simulink model "Advance Traction Motor and Regeneration Modeling"  (R2021a)
settings: Solver=FixedStepAuto  StartTime=0.0  StopTime=inf  FixedStep=1  RelTol=1e-3
values from neighbouring files (symbols this model uses):
  Battery_E = 24000    [Imports.m]
  BPC = 66.2    [Imports.m]
  C_SOC = Value3(:,3)    [Imports.m]
  C_V = Value3(:,2)    [Imports.m]
  Cd = 0.28    [Imports.m]
  Crf = 0.015    [Imports.m]
  Fa = 3.8056    [Imports.m]
  GR = 7.9377    [Imports.m]
  GVM = Mv+Md    (= 1710.665)    [Imports.m]
  GVW = GVM*g    (= 16781.62365)    [Imports.m]
  Ir = 0.0023    [Imports.m]
  Kemf = 0.238    [Imports.m]
  Kt = 0.195    [Imports.m]
  LSOC = 20    [Imports.m]
  M_B_R_C = M_R_C*Np    (= 66.2)    [Imports.m]
  Ns = 96    [Imports.m]
  Ra = 0.00567    [Imports.m]
  rho = 1.225    [Imports.m]
  Rw = 0.2032    [Imports.m]
  Teff = 0.89    [Imports.m]
  USOC = 80    [Imports.m]
undefined symbols (not defined in the file or in its folder): NL_M, NL_MC, NL_RM
settings Model: Creator=goodbox  LastModifiedBy=LENOVO
settings SolverCC: ShapePreserveControl=EnableAll  AlgebraicLoopSolver=TrustRegion
settings DebuggingCC: SFMachineParentedDataDiag=warning

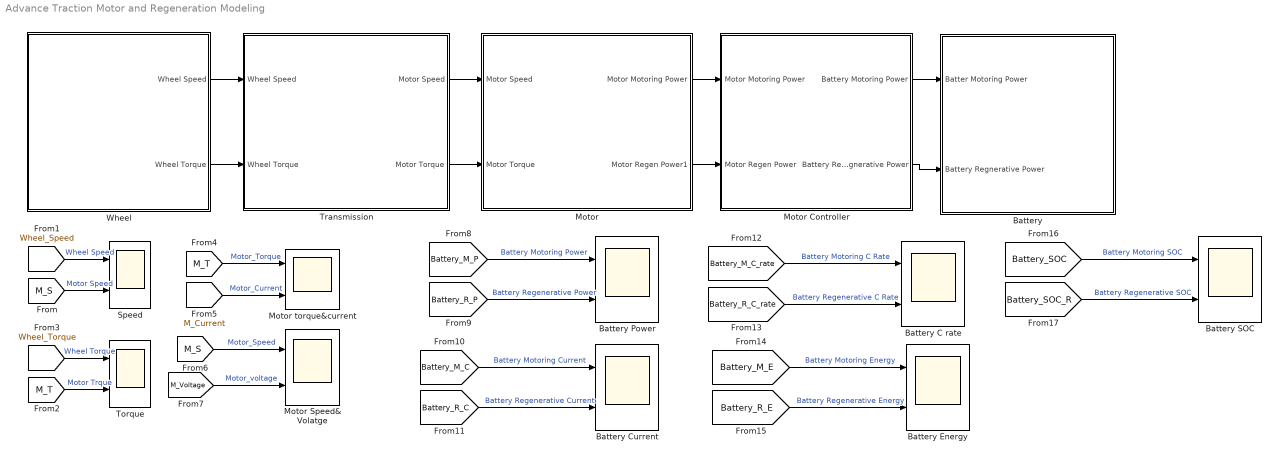
== system Advance Traction Motor and Regeneration Modeling ==
  Battery : Subsystem
  Battery C rate : Scope  NumInputPorts=2
  Battery Current : Scope  NumInputPorts=2
  Battery Energy : Scope  NumInputPorts=2
  Battery Power : Scope  NumInputPorts=2
  Battery SOC : Scope  NumInputPorts=2
  Motor : Subsystem
  Motor Controller : Subsystem
  Motor Speed& Volatge : Scope  NumInputPorts=2
  Motor torque&current : Scope  NumInputPorts=2
  Speed : Scope  NumInputPorts=2
  Torque : Scope  NumInputPorts=2
  Transmission : Subsystem
  Wheel : Subsystem
  wires:
  Wheel/1(Wheel Speed) -> Transmission/1(Wheel Speed)
  Wheel/2(Wheel Torque) -> Transmission/2(Wheel Torque)
  [Wheel_Speed] -> Speed/1  "Wheel Speed"
  [M_S] -> Speed/2  "Motor Speed"
  [M_T] -> Torque/2  "Motor Trque"
  [Wheel_Torque] -> Torque/1  "Wheel Torque"
  Transmission/1(Motor Speed) -> Motor/1(Motor Speed)
  Transmission/2(Motor Torque) -> Motor/2(Motor Torque)
  [M_T] -> Motor torque&current/1  "Motor_Torque"
  [M_Current] -> Motor torque&current/2  "Motor_Current"
  [M_S] -> Motor Speed& Volatge/1  "Motor_Speed"
  [M_Voltage] -> Motor Speed& Volatge/2  "Motor_voltage"
  Motor/1(Motor Motoring Power) -> Motor Controller/1(Motor Motoring Power)
  Motor/2(Motor Regen Power1) -> Motor Controller/2(Motor Regen Power)
  Motor Controller/1(Battery Motoring Power) -> Battery/1(Batter Motoring Power)
  Motor Controller/2(Battery Regnerative Power) -> Battery/2(Battery Regnerative Power)
  [Battery_M_P] -> Battery Power/1  "Battery Motoring Power"
  [Battery_R_P] -> Battery Power/2  "Battery Regenerative Power"
  [Battery_R_C] -> Battery Current/2  "Battery Regenerative Current"
  [Battery_M_C] -> Battery Current/1  "Battery Motoring Current"
  [Battery_M_C_rate] -> Battery C rate/1  "Battery Motoring C Rate"
  [Battery_R_C_rate] -> Battery C rate/2  "Battery Regenerative C Rate"
  [Battery_M_E] -> Battery Energy/1  "Battery Motoring Energy"
  [Battery_R_E] -> Battery Energy/2  "Battery Regenerative Energy"
  [Battery_SOC_R] -> Battery SOC/2  "Battery Regenerative SOC"
  [Battery_SOC] -> Battery SOC/1  "Battery Motoring SOC"

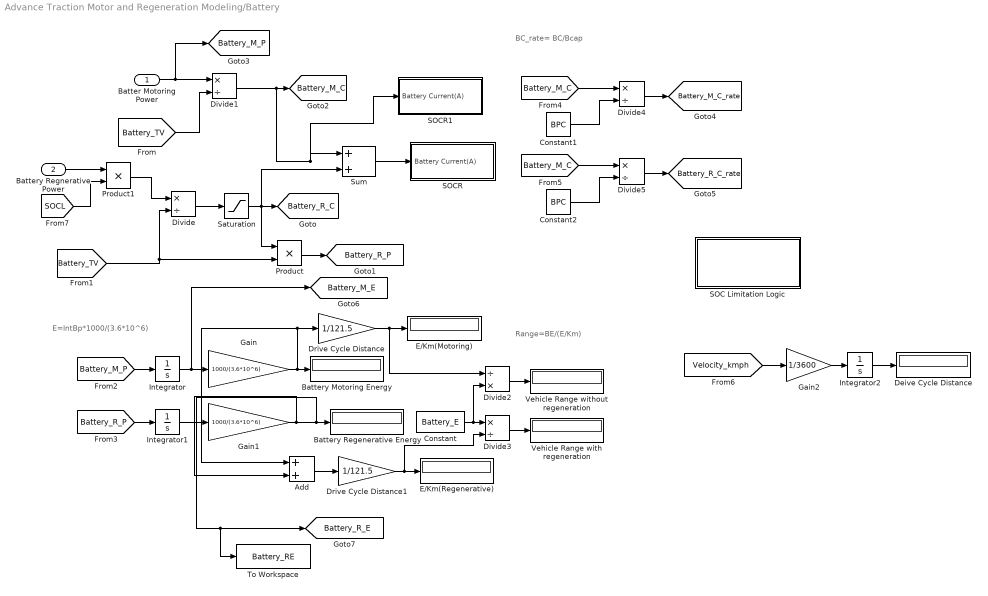
== system Advance Traction Motor and Regeneration Modeling/Battery ==
  note: BC_rate= BC/Bcap
  note: Range=BE/(E/Km)
  note: E=IntBp*1000/(3.6*10^6)
  Batter Motoring Power : Inport
  Battery Regnerative Power : Inport  Port=2
  Add : Sum
  Battery Motoring Energy : Display
  Battery Regenerative Energy : Display
  Constant : Constant  Value=Battery_E
  Constant1 : Constant  Value=BPC
  Constant2 : Constant  Value=BPC
  Deive Cycle Distance : Display
  Divide{,1,3..5} (5 alike) : Product  Inputs=*/
  Divide2 : Product  Inputs=/*
  Drive Cycle Distance : Gain  Gain=1/121.5
  Drive Cycle Distance1 : Gain  Gain=1/121.5
  E/Km(Motoring) : Display
  E/Km(Regenerative) : Display
  Gain : Gain  Gain=1000/(3.6*10^6)
  Gain1 : Gain  Gain=1000/(3.6*10^6)
  Gain2 : Gain  Gain=1/3600
  Integrator : Integrator
  Integrator1 : Integrator
  Integrator2 : Integrator
  Product : Product
  Product1 : Product
  SOC Limitation Logic : Subsystem
  SOCR : Subsystem
  SOCR1 : Subsystem
  Saturation : Saturate  UpperLimit=0  LowerLimit=-M_B_R_C
  Sum : Sum  Inputs=|++
  To Workspace : ToWorkspace  VariableName=Battery_RE  SaveFormat=Timeseries  SampleTime=-1
  Vehicle Range with regeneration : Display
  Vehicle Range without regeneration : Display
  tag scope: Battery_M_C=global, Battery_M_C_rate=global, Battery_M_E=global, Battery_M_P=global, Battery_R_C=global, Battery_R_C_rate=global, Battery_R_E=global, Battery_R_P=global
  wires:
  [Battery_TV] -> Divide/2, Product/2
  Divide/1 -> Saturation/1
  Saturation/1 -> Sum/2, Product/1, [Battery_R_C]
  Product/1 -> [Battery_R_P]
  Batter Motoring Power/1 -> [Battery_M_P], Divide1/1
  [Battery_TV] -> Divide1/2
  Divide1/1 -> SOCR1/1("Battery Current(A) "), Sum/1, [Battery_M_C]
  Sum/1 -> SOCR/1("Battery Current(A) ")
  [Battery_M_P] -> Integrator/1
  Integrator/1 -> [Battery_M_E], Gain/1
  Gain/1 -> Add/1, Drive Cycle Distance/1, Battery Motoring Energy/1
  [Battery_R_P] -> Integrator1/1
  Integrator1/1 -> Gain1/1
  Drive Cycle Distance/1 -> Divide2/1, E/Km(Motoring)/1
  Gain1/1 -> Add/2, To Workspace/1, [Battery_R_E], Battery Regenerative Energy/1
  Drive Cycle Distance1/1 -> Divide3/2, E/Km(Regenerative)/1
  Add/1 -> Drive Cycle Distance1/1
  Constant/1 -> Divide3/1, Divide2/2
  Divide3/1 -> Vehicle Range with regeneration/1
  Divide2/1 -> Vehicle Range without regeneration/1
  [Battery_M_C] -> Divide4/1
  Constant1/1 -> Divide4/2
  Divide4/1 -> [Battery_M_C_rate]
  Divide5/1 -> [Battery_R_C_rate]
  Constant2/1 -> Divide5/2
  [Battery_M_C] -> Divide5/1
  [Velocity_kmph] -> Gain2/1
  Gain2/1 -> Integrator2/1
  Integrator2/1 -> Deive Cycle Distance/1
  Battery Regnerative Power/1 -> Product1/1
  [SOCL] -> Product1/2
  Product1/1 -> Divide/1

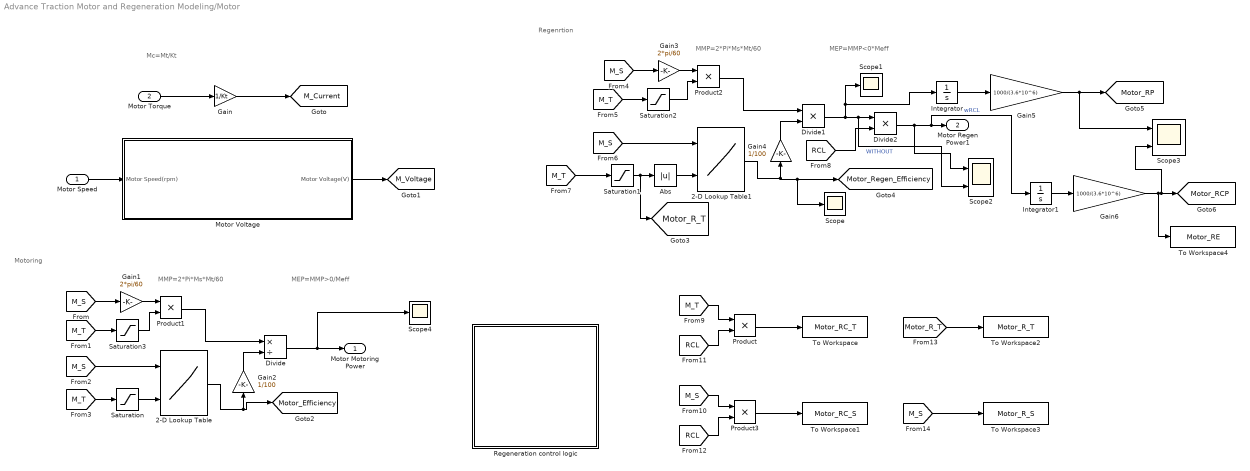
== system Advance Traction Motor and Regeneration Modeling/Motor ==
  note: Regenrtion
  note: MEP=MMP>0/Meff
  note: MMP=2*Pi*Ms*Mt/60
  note: Motoring
  note: Mc=Mt/Kt
  note: MEP=MMP<0*Meff
  note: MMP=2*Pi*Ms*Mt/60
  Motor Speed : Inport
  Motor Torque : Inport  Port=2
  2-D Lookup Table : Lookup_n-D  BreakpointsForDimension1=NL_M.Speed  BreakpointsForDimension2=NL_M.Torque  Table=NL_M.Efficiency  InternalRulePriority=Speed  RndMeth=Simplest  InputSameDT=on
      settings: InputPortMap=u0,u1
  2-D Lookup Table1 : Lookup_n-D  BreakpointsForDimension1=NL_RM.Speed  BreakpointsForDimension2=NL_RM.Torque  Table=NL_RM.Efficiency  InternalRulePriority=Speed  RndMeth=Simplest  InputSameDT=on
      settings: InputPortMap=u0,u1
  Abs : Abs
  Divide : Product  Inputs=*/
  Divide1 : Product  Inputs=**
  Divide2 : Product  Inputs=**
  Gain : Gain  Gain=1/Kt
  Gain1 : Gain  Gain=2*pi/60
  Gain2 : Gain  Gain=1/100
  Gain3 : Gain  Gain=2*pi/60
  Gain4 : Gain  Gain=1/100
  Gain5 : Gain  Gain=1000/(3.6*10^6)
  Gain6 : Gain  Gain=1000/(3.6*10^6)
  Integrator : Integrator
  Integrator1 : Integrator
  Motor Voltage : Subsystem
  Product{,1..3} (4 alike) : Product
  Regeneration control logic : Subsystem
  Saturation : Saturate  UpperLimit=inf  LowerLimit=0
  Saturation1 : Saturate  UpperLimit=0  LowerLimit=-inf
  Saturation2 : Saturate  UpperLimit=0  LowerLimit=-inf
  Saturation3 : Saturate  UpperLimit=inf  LowerLimit=0
  Scope : Scope
  Scope1 : Scope
  Scope2 : Scope  NumInputPorts=2
  Scope3 : Scope  NumInputPorts=2
  Scope4 : Scope
  To Workspace : ToWorkspace  VariableName=Motor_RC_T  SaveFormat=Timeseries  SampleTime=-1
  To Workspace1 : ToWorkspace  VariableName=Motor_RC_S  SaveFormat=Timeseries  SampleTime=-1
  To Workspace2 : ToWorkspace  VariableName=Motor_R_T  SaveFormat=Timeseries  SampleTime=-1
  To Workspace3 : ToWorkspace  VariableName=Motor_R_S  SaveFormat=Timeseries  SampleTime=-1
  To Workspace4 : ToWorkspace  VariableName=Motor_RE  SaveFormat=Timeseries  SampleTime=-1
  Motor Motoring Power : Outport
  Motor Regen Power1 : Outport  Port=2
  tag scope: M_Current=global, M_Voltage=global, Motor_Efficiency=global, Motor_RCP=global, Motor_RP=global, Motor_R_T=global, Motor_Regen_Efficiency=global
  wires:
  Motor Torque/1 -> Gain/1
  Gain/1 -> [M_Current]
  Motor Speed/1 -> Motor Voltage/1(Motor Speed(rpm))
  Motor Voltage/1(Motor Voltage(V)) -> [M_Voltage]
  [M_S] -> Gain1/1
  Gain1/1 -> Product1/1
  [M_T] -> Saturation3/1
  [M_S] -> 2-D Lookup Table/1
  [M_T] -> Saturation/1
  Product1/1 -> Divide/1
  2-D Lookup Table/1 -> Gain2/1, [Motor_Efficiency]
  Gain2/1 -> Divide/2
  Divide/1 -> Scope4/1, Motor Motoring Power/1
  Gain4/1 -> Divide1/2
  2-D Lookup Table1/1 -> Gain4/1, Scope/1, [Motor_Regen_Efficiency]
  [M_T] -> Saturation1/1
  Product2/1 -> Divide1/1
  Gain3/1 -> Product2/1
  [M_S] -> Gain3/1
  [M_S] -> 2-D Lookup Table1/1
  [M_T] -> Saturation2/1
  Saturation1/1 -> [Motor_R_T], Abs/1
  Abs/1 -> 2-D Lookup Table1/2
  Saturation2/1 -> Product2/2
  Saturation/1 -> 2-D Lookup Table/2
  Saturation3/1 -> Product1/2
  Divide1/1 -> Scope2/2, Divide2/1, Integrator/1, Scope1/1  "WITHOUT"
  Divide2/1 -> Scope2/1, Integrator1/1, Motor Regen Power1/1  "wRCL"
  [RCL] -> Divide2/2
  Gain5/1 -> Scope3/1, [Motor_RP]
  Integrator/1 -> Gain5/1
  Gain6/1 -> [Motor_RCP], Scope3/2, To Workspace4/1
  Integrator1/1 -> Gain6/1
  [M_T] -> Product/1
  [RCL] -> Product3/2
  [M_S] -> Product3/1
  [RCL] -> Product/2
  Product/1 -> To Workspace/1
  Product3/1 -> To Workspace1/1
  [Motor_R_T] -> To Workspace2/1
  [M_S] -> To Workspace3/1

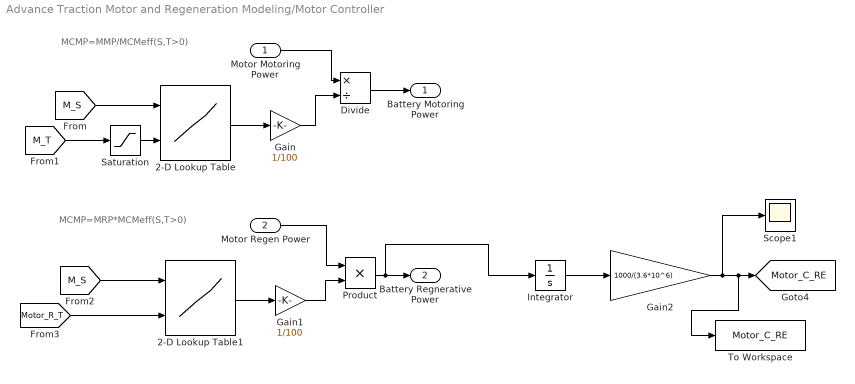
== system Advance Traction Motor and Regeneration Modeling/Motor Controller ==
  note: MCMP=MMP/MCMeff(S,T>0)
  note: MCMP=MRP*MCMeff(S,T>0)
  Motor Motoring Power : Inport
  Motor Regen Power : Inport  Port=2
  2-D Lookup Table : Lookup_n-D  BreakpointsForDimension1=NL_MC.Speed  BreakpointsForDimension2=NL_MC.Torque  Table=NL_MC.Efficiency  InternalRulePriority=Speed  RndMeth=Simplest  InputSameDT=on
      settings: InputPortMap=u0,u1
  2-D Lookup Table1 : Lookup_n-D  BreakpointsForDimension1=NL_MC.Speed  BreakpointsForDimension2=NL_MC.Torque  Table=NL_MC.Efficiency  InternalRulePriority=Speed  RndMeth=Simplest  InputSameDT=on
      settings: InputPortMap=u0,u1
  Divide : Product  Inputs=*/
  Gain : Gain  Gain=1/100
  Gain1 : Gain  Gain=1/100
  Gain2 : Gain  Gain=1000/(3.6*10^6)
  Integrator : Integrator
  Product : Product
  Saturation : Saturate  UpperLimit=inf  LowerLimit=0
  Scope1 : Scope
  To Workspace : ToWorkspace  VariableName=Motor_C_RE  SaveFormat=Timeseries  SampleTime=-1
  Battery Motoring Power : Outport
  Battery Regnerative Power : Outport  Port=2
  tag scope: Motor_C_RE=global
  wires:
  [M_S] -> 2-D Lookup Table/1
  Saturation/1 -> 2-D Lookup Table/2
  [M_T] -> Saturation/1
  2-D Lookup Table/1 -> Gain/1
  Motor Motoring Power/1 -> Divide/1
  Gain/1 -> Divide/2
  Divide/1 -> Battery Motoring Power/1
  [Motor_R_T] -> 2-D Lookup Table1/2
  Motor Regen Power/1 -> Product/1
  [M_S] -> 2-D Lookup Table1/1
  2-D Lookup Table1/1 -> Gain1/1
  Gain1/1 -> Product/2
  Product/1 -> Integrator/1, Battery Regnerative Power/1
  Integrator/1 -> Gain2/1
  Gain2/1 -> Scope1/1, To Workspace/1, [Motor_C_RE]

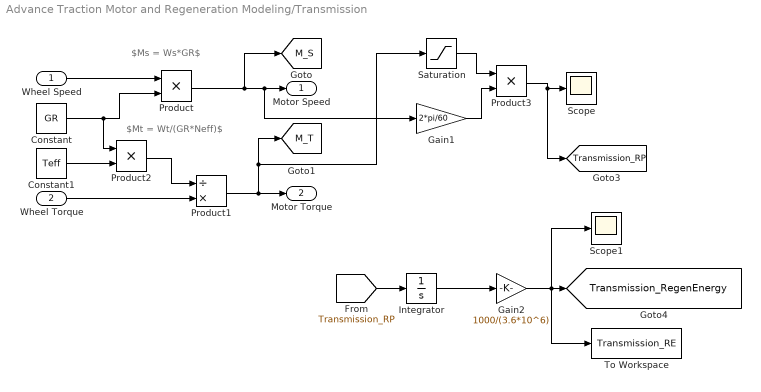
== system Advance Traction Motor and Regeneration Modeling/Transmission ==
  note: $Mt = Wt/(GR*Neff)$
  note: $Ms = Ws*GR$
  Wheel Speed : Inport
  Wheel Torque : Inport  Port=2
  Constant : Constant  Value=GR
  Constant1 : Constant  Value=Teff
  Gain1 : Gain  Gain=2*pi/60
  Gain2 : Gain  Gain=1000/(3.6*10^6)
  Integrator : Integrator
  Product : Product
  Product1 : Product  Inputs=/*
  Product2 : Product
  Product3 : Product
  Saturation : Saturate  UpperLimit=0  LowerLimit=-inf
  Scope : Scope
  Scope1 : Scope
  To Workspace : ToWorkspace  VariableName=Transmission_RE  SaveFormat=Timeseries  SampleTime=-1
  Motor Speed : Outport
  Motor Torque : Outport  Port=2
  tag scope: M_S=global, M_T=global, Transmission_RP=global, Transmission_RegenEnergy=global
  wires:
  Wheel Speed/1 -> Product/1
  Constant/1 -> Product2/1, Product/2
  Constant1/1 -> Product2/2
  Wheel Torque/1 -> Product1/2
  Product2/1 -> Product1/1
  Integrator/1 -> Gain2/1
  Gain2/1 -> To Workspace/1, Scope1/1, [Transmission_RegenEnergy]
  Product1/1 -> Saturation/1, [M_T], Motor Torque/1
  Product/1 -> [M_S], Gain1/1, Motor Speed/1
  Saturation/1 -> Product3/1
  Product3/1 -> [Transmission_RP], Scope/1
  Gain1/1 -> Product3/2
  [Transmission_RP] -> Integrator/1

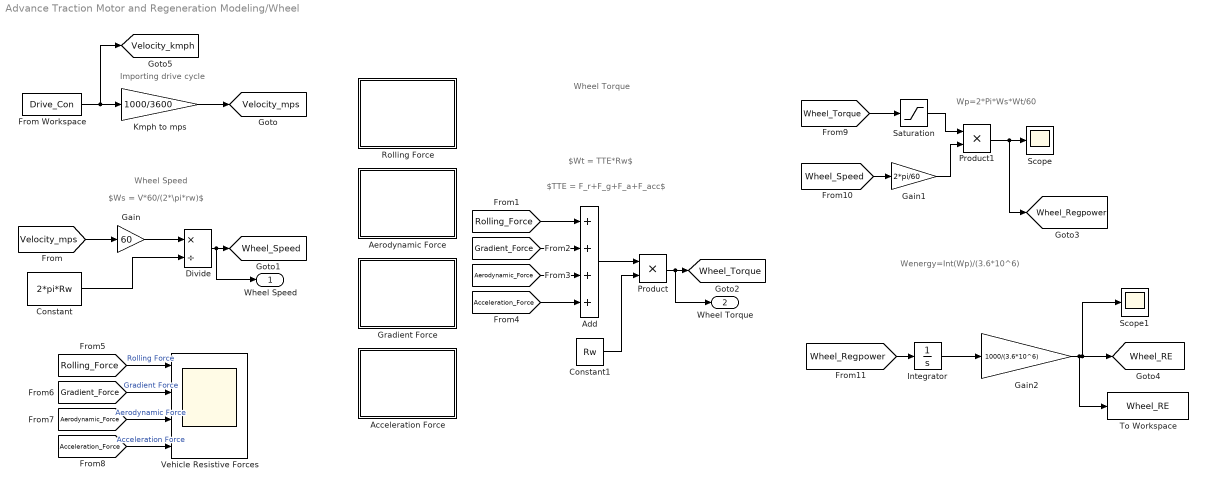
== system Advance Traction Motor and Regeneration Modeling/Wheel ==
  note: Wenergy=Int(Wp)/(3.6*10^6)
  note: Wp=2*Pi*Ws*Wt/60
  note: $TTE = F_r+F_g+F_a+F_acc$
  note: $Wt = TTE*Rw$
  note: Wheel Torque
  note: $Ws = V*60/(2*\pi*rw)$
  note: Wheel Speed
  note: Importing drive cycle
  Acceleration Force : Subsystem
  Add : Sum  Inputs=4
  Aerodynamic Force : Subsystem
  Constant : Constant  Value=2*pi*Rw
  Constant1 : Constant  Value=Rw
  Divide : Product  Inputs=*/
  From Workspace : FromWorkspace  VariableName=Drive_Con
  Gain : Gain  Gain=60
  Gain1 : Gain  Gain=2*pi/60
  Gain2 : Gain  Gain=1000/(3.6*10^6)
  Gradient Force : Subsystem
  Integrator : Integrator
  Kmph to mps : Gain  Gain=1000/3600
  Product : Product
  Product1 : Product
  Rolling Force : Subsystem
  Saturation : Saturate  UpperLimit=0  LowerLimit=-inf
  Scope : Scope
  Scope1 : Scope
  To Workspace : ToWorkspace  VariableName=Wheel_RE  SaveFormat=Timeseries  SampleTime=-1
  Vehicle Resistive Forces : Scope  NumInputPorts=4
  Wheel Speed : Outport
  Wheel Torque : Outport  Port=2
  tag scope: Velocity_kmph=global, Velocity_mps=global, Wheel_RE=global, Wheel_Regpower=global, Wheel_Speed=global, Wheel_Torque=global
  wires:
  From Workspace/1 -> [Velocity_kmph], Kmph to mps/1
  Kmph to mps/1 -> [Velocity_mps]
  [Velocity_mps] -> Gain/1
  Gain/1 -> Divide/1
  Constant/1 -> Divide/2
  Divide/1 -> Wheel Speed/1, [Wheel_Speed]
  [Rolling_Force] -> Add/1
  [Gradient_Force] -> Add/2
  [Aerodynamic_Force] -> Add/3
  [Acceleration_Force] -> Add/4
  Add/1 -> Product/1
  Constant1/1 -> Product/2
  Product/1 -> Wheel Torque/1, [Wheel_Torque]
  [Rolling_Force] -> Vehicle Resistive Forces/1  "Rolling Force"
  [Gradient_Force] -> Vehicle Resistive Forces/2  "Gradient Force"
  [Aerodynamic_Force] -> Vehicle Resistive Forces/3  "Aerodynamic Force"
  [Acceleration_Force] -> Vehicle Resistive Forces/4  "Acceleration Force"
  [Wheel_Torque] -> Saturation/1
  [Wheel_Speed] -> Gain1/1
  Saturation/1 -> Product1/1
  Gain1/1 -> Product1/2
  Product1/1 -> [Wheel_Regpower], Scope/1
  [Wheel_Regpower] -> Integrator/1
  Integrator/1 -> Gain2/1
  Gain2/1 -> To Workspace/1, Scope1/1, [Wheel_RE]

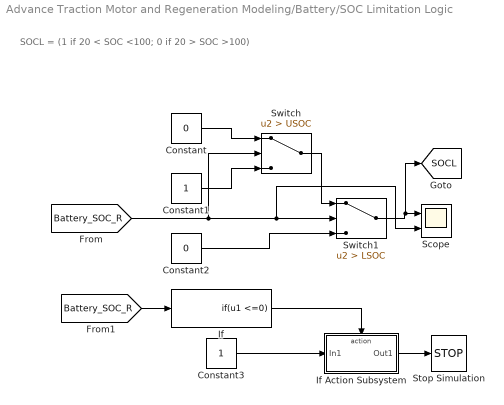
== system Advance Traction Motor and Regeneration Modeling/Battery/SOC Limitation Logic ==
  note: SOCL = (1 if 20 < SOC <100; 0 if 20 > SOC >100)
  Constant : Constant  Value=0
  Constant1 : Constant
  Constant2 : Constant  Value=0
  Constant3 : Constant
  If : If  IfExpression=u1 <=0  ShowElse=off
  If Action Subsystem : Subsystem  TreatAsAtomicUnit=on
  Scope : Scope  NumInputPorts=2
  Stop Simulation : Stop
  Switch : Switch  Criteria=u2 > Threshold  Threshold=USOC
  Switch1 : Switch  Criteria=u2 > Threshold  Threshold=LSOC
  tag scope: SOCL=global
  wires:
  Constant/1 -> Switch/1
  Constant1/1 -> Switch/3
  [Battery_SOC_R] -> Switch/2, Scope/2, Switch1/2
  Constant2/1 -> Switch1/3
  Switch/1 -> Switch1/1
  Switch1/1 -> [SOCL], Scope/1
  [Battery_SOC_R] -> If/1
  Constant3/1 -> If Action Subsystem/1(In1)
  If/1 -> If Action Subsystem/Action
  If Action Subsystem/1(Out1) -> Stop Simulation/1

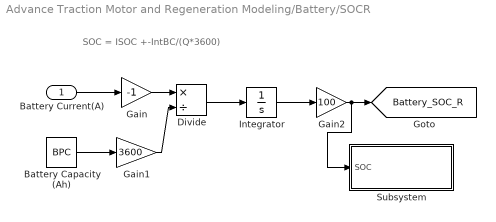
== system Advance Traction Motor and Regeneration Modeling/Battery/SOCR ==
  note: SOC = ISOC +-IntBC/(Q*3600)
  "Battery Current(A) " : Inport
  Battery Capacity (Ah) : Constant  Value=BPC
  Divide : Product  Inputs=*/
  Gain : Gain  Gain=-1
  Gain1 : Gain  Gain=3600
  Gain2 : Gain  Gain=100
  Integrator : Integrator  InitialCondition=1
  Subsystem : Subsystem
  tag scope: Battery_SOC_R=global
  wires:
  "Battery Current(A) "/1 -> Gain/1
  Battery Capacity (Ah)/1 -> Gain1/1
  Gain/1 -> Divide/1
  Gain1/1 -> Divide/2
  Divide/1 -> Integrator/1
  Integrator/1 -> Gain2/1
  Gain2/1 -> Subsystem/1(SOC), [Battery_SOC_R]

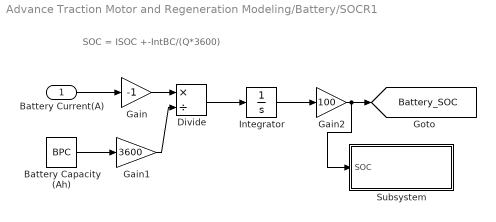
== system Advance Traction Motor and Regeneration Modeling/Battery/SOCR1 ==
  note: SOC = ISOC +-IntBC/(Q*3600)
  "Battery Current(A) " : Inport
  Battery Capacity (Ah) : Constant  Value=BPC
  Divide : Product  Inputs=*/
  Gain : Gain  Gain=-1
  Gain1 : Gain  Gain=3600
  Gain2 : Gain  Gain=100
  Integrator : Integrator  InitialCondition=1
  Subsystem : Subsystem
  tag scope: Battery_SOC=global
  wires:
  "Battery Current(A) "/1 -> Gain/1
  Battery Capacity (Ah)/1 -> Gain1/1
  Gain/1 -> Divide/1
  Gain1/1 -> Divide/2
  Divide/1 -> Integrator/1
  Integrator/1 -> Gain2/1
  Gain2/1 -> Subsystem/1(SOC), [Battery_SOC]

== system Advance Traction Motor and Regeneration Modeling/Motor/Motor Voltage ==
  note: Mv=Ms*Kemf+I*Ra
  Motor Speed(rpm) : Inport
  Add : Sum
  Gain : Gain  Gain=Ra
  Saturation : Saturate  UpperLimit=inf  LowerLimit=0
  Volts : Gain  Gain=Kemf
  rpm to rad/s : Gain  Gain=2*pi/60
  Motor Voltage(V) : Outport
  wires:
  Motor Speed(rpm)/1 -> rpm to rad/s/1
  rpm to rad/s/1 -> Volts/1  "rad/s"
  [M_Current] -> Gain/1
  Volts/1 -> Add/1
  Gain/1 -> Add/2
  Add/1 -> Saturation/1
  Saturation/1 -> Motor Voltage(V)/1

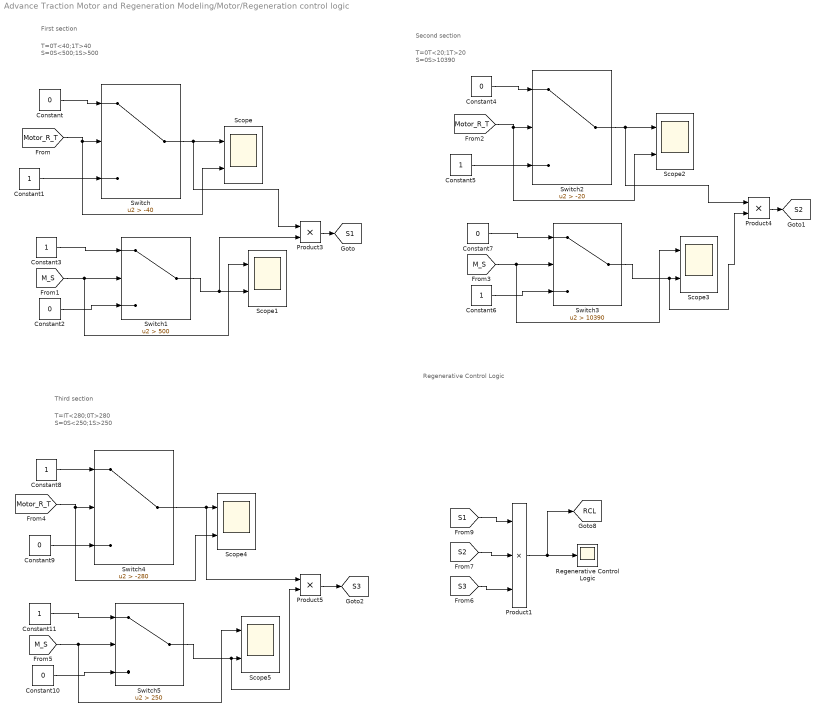
== system Advance Traction Motor and Regeneration Modeling/Motor/Regeneration control logic ==
  note: T=0T<40;1T>40
      | S=0S<500;1S>500
  note: First section
  note: T=0T<20;1T>20
      | S=0S>10390
  note: Second section
  note: Third section
  note: T=IT<280;0T>280
      | S=0S<250;1S>250
  note: Regenerative Control Logic
  Constant{,2,4,7,9..10} (6 alike) : Constant  Value=0
  Constant{1,3,5..6,8,11} (6 alike) : Constant
  Product1 : Product  Inputs=3
  Product3 : Product
  Product4 : Product
  Product5 : Product
  Regenerative	Control Logic : Scope
  Scope{,1..5} (6 alike) : Scope  NumInputPorts=2
  Switch : Switch  Criteria=u2 > Threshold  Threshold=-40
  Switch1 : Switch  Criteria=u2 > Threshold  Threshold=500
  Switch2 : Switch  Criteria=u2 > Threshold  Threshold=-20
  Switch3 : Switch  Criteria=u2 > Threshold  Threshold=10390
  Switch4 : Switch  Criteria=u2 > Threshold  Threshold=-280
  Switch5 : Switch  Criteria=u2 > Threshold  Threshold=250
  tag scope: RCL=global, S1=global, S2=global, S3=global
  wires:
  [Motor_R_T] -> Scope/2, Switch/2
  Constant/1 -> Switch/1
  Constant1/1 -> Switch/3
  Switch/1 -> Product3/1, Scope/1
  [M_S] -> Scope1/1, Switch1/2
  Constant3/1 -> Switch1/1
  Constant2/1 -> Switch1/3
  Switch1/1 -> Product3/2, Scope1/2
  [M_S] -> Scope3/1, Switch3/2
  Switch3/1 -> Product4/2, Scope3/2
  Switch2/1 -> Product4/1, Scope2/1
  Constant6/1 -> Switch3/3
  Constant7/1 -> Switch3/1
  [Motor_R_T] -> Scope2/2, Switch2/2
  Constant5/1 -> Switch2/3
  Constant4/1 -> Switch2/1
  [M_S] -> Scope5/1, Switch5/2
  Switch5/1 -> Product5/2, Scope5/2
  Constant10/1 -> Switch5/3
  Constant11/1 -> Switch5/1
  [Motor_R_T] -> Scope4/2, Switch4/2
  Constant9/1 -> Switch4/3
  Constant8/1 -> Switch4/1
  [S1] -> Product1/1
  [S2] -> Product1/2
  [S3] -> Product1/3
  Product1/1 -> [RCL], Regenerative	Control Logic/1
  Product3/1 -> [S1]
  Product4/1 -> [S2]
  Product5/1 -> [S3]
  Switch4/1 -> Product5/1, Scope4/1

== system Advance Traction Motor and Regeneration Modeling/Wheel/Acceleration Force ==
  note: $Facc = GVM*a$
  Constant : Constant  Value=GVM
  Derivative : Derivative
  Product : Product
  tag scope: Acceleration_Force=global
  wires:
  [Velocity_mps] -> Derivative/1
  Constant/1 -> Product/1
  Derivative/1 -> Product/2
  Product/1 -> [Acceleration_Force]

== system Advance Traction Motor and Regeneration Modeling/Wheel/Aerodynamic Force ==
  note: $Fa = 0.5*rho*Fa*Cd*V^2$
  Air density : Constant  Value=rho
  Constant : Constant  Value=0.5
  Drag coefficient : Constant  Value=Cd
  Frontal Area : Constant  Value=Fa
  Product : Product  Inputs=5
  Square : Math  Operator=square  SaturateOnIntegerOverflow=on
  tag scope: Aerodynamic_Force=global
  wires:
  [Velocity_mps] -> Square/1
  Square/1 -> Product/5
  Drag coefficient/1 -> Product/4
  Frontal Area/1 -> Product/3
  Air density/1 -> Product/2
  Constant/1 -> Product/1
  Product/1 -> [Aerodynamic_Force]

== system Advance Traction Motor and Regeneration Modeling/Wheel/Gradient Force ==
  note: $Fg = GVW*sin(\theta)$
  Constant : Constant  Value=GVW
  Gain : Gain  Gain=pi/180
  Grade angle : Constant  Value=0
  Product : Product
  Sin : Trigonometry
  tag scope: Gradient_Force=global
  wires:
  Grade angle/1 -> Gain/1
  Gain/1 -> Sin/1
  Constant/1 -> Product/1
  Sin/1 -> Product/2
  Product/1 -> [Gradient_Force]

== system Advance Traction Motor and Regeneration Modeling/Wheel/Rolling Force ==
  note: $Fr = GVW*Crf$
  Constant : Constant  Value=GVW
  Constant1 : Constant  Value=Crf
  Product : Product
  tag scope: Rolling_Force=global
  wires:
  Constant/1 -> Product/1
  Constant1/1 -> Product/2
  Product/1 -> [Rolling_Force]

== system Advance Traction Motor and Regeneration Modeling/Battery/SOC Limitation Logic/If Action Subsystem ==
  In1 : Inport
  Action Port : ActionPort  ActionPortLabel=if(u1 <=0)
  Out1 : Outport
  wires:
  In1/1 -> Out1/1

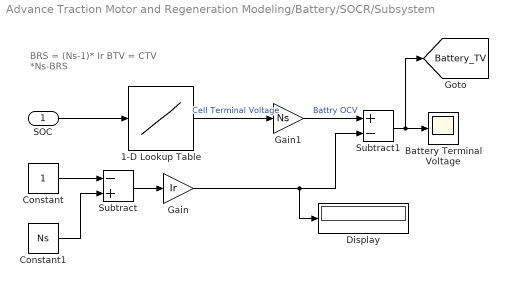
== system Advance Traction Motor and Regeneration Modeling/Battery/SOCR/Subsystem ==
  note: BRS = (Ns-1)* Ir
      | BTV = CTV *Ns-BRS
  SOC : Inport
  1-D Lookup Table : Lookup_n-D  NumberOfTableDimensions=1  BreakpointsForDimension1=C_SOC  Table=C_V  InternalRulePriority=Speed  RndMeth=Simplest  InputSameDT=on
  Battery Terminal Voltage : Scope
  Constant : Constant
  Constant1 : Constant  Value=Ns
  Display : Display
  Gain : Gain  Gain=Ir
  Gain1 : Gain  Gain=Ns
  Subtract : Sum  Inputs=-+
  Subtract1 : Sum  Inputs=+-
  tag scope: Battery_TV=global
  wires:
  Constant/1 -> Subtract/1
  Constant1/1 -> Subtract/2
  Subtract/1 -> Gain/1
  SOC/1 -> 1-D Lookup Table/1
  1-D Lookup Table/1 -> Gain1/1  "Cell Terminal Voltage"
  Gain1/1 -> Subtract1/1  "Battry OCV"
  Gain/1 -> Display/1, Subtract1/2
  Subtract1/1 -> [Battery_TV], Battery Terminal Voltage/1

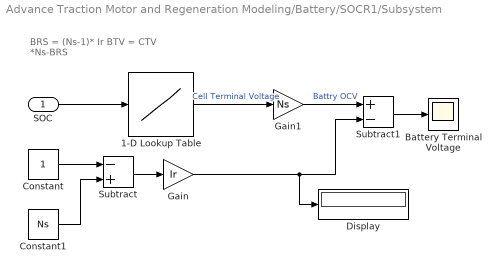
== system Advance Traction Motor and Regeneration Modeling/Battery/SOCR1/Subsystem ==
  note: BRS = (Ns-1)* Ir
      | BTV = CTV *Ns-BRS
  SOC : Inport
  1-D Lookup Table : Lookup_n-D  NumberOfTableDimensions=1  BreakpointsForDimension1=C_SOC  Table=C_V  InternalRulePriority=Speed  RndMeth=Simplest  InputSameDT=on
  Battery Terminal Voltage : Scope
  Constant : Constant
  Constant1 : Constant  Value=Ns
  Display : Display
  Gain : Gain  Gain=Ir
  Gain1 : Gain  Gain=Ns
  Subtract : Sum  Inputs=-+
  Subtract1 : Sum  Inputs=+-
  wires:
  Constant/1 -> Subtract/1
  Constant1/1 -> Subtract/2
  Subtract/1 -> Gain/1
  SOC/1 -> 1-D Lookup Table/1
  1-D Lookup Table/1 -> Gain1/1  "Cell Terminal Voltage"
  Gain1/1 -> Subtract1/1  "Battry OCV"
  Gain/1 -> Display/1, Subtract1/2
  Subtract1/1 -> Battery Terminal Voltage/1
